simulink model "station_no_recovery"  (R2015a)
settings: Solver=ode45  StartTime=0  StopTime=5000  FixedStep=10  MaxStep=1  RelTol=1e-3
(part 4 of 4)

== system station_no_recovery/Восстанавливаемые объекты/ПАЭС-2500/Subsystem2/Element Exponential1 ==
  note: интенсивность событий
      | в рассматриваемом потоке
  "lambda " : Inport
  t : Inport  Port=2
  Divide : Product  Inputs=**
  Gain : Gain  Gain=-1
  Math Function : Math  SaturateOnIntegerOverflow=on
  P(t)1 : Outport
  wires:
  "lambda "/1 -> Divide/2
  Math Function/1 -> P(t)1/1
  Gain/1 -> Math Function/1
  t/1 -> Divide/1
  Divide/1 -> Gain/1

== system station_no_recovery/Восстанавливаемые объекты/ПАЭС-2500/Subsystem2/Element Normal ==
  note: математическое ожидание
      | наработки до отказа
  note: среднее квадратическое
      | отклонение наработки
      | до отказа
  "lambda " : Inport
  "M " : Inport  Port=2
  t : Inport  Port=3
  1-Q(t)1 : Fcn  Expr=1-u(1)
  MATLAB Function : MATLAB Function  TreatAsAtomicUnit=on
  P(t) : Outport
  wires:
  t/1 -> MATLAB Function/1(t)
  MATLAB Function/1(y) -> 1-Q(t)1/1
  "lambda "/1 -> MATLAB Function/2(sigma)
  1-Q(t)1/1 -> P(t)/1
  "M "/1 -> MATLAB Function/3(M)

== system station_no_recovery/Восстанавливаемые объекты/ПАЭС-2500/Subsystem2/Element Normal1 ==
  note: среднее квадратическое
      | отклонение наработки
      | до отказа
  note: математическое ожидание
      | наработки до отказа
  "lambda " : Inport
  "M " : Inport  Port=2
  t : Inport  Port=3
  1-Q(t)1 : Fcn  Expr=1-u(1)
  MATLAB Function : MATLAB Function  TreatAsAtomicUnit=on
  P(t) : Outport
  wires:
  "M "/1 -> MATLAB Function/3(M)
  1-Q(t)1/1 -> P(t)/1
  "lambda "/1 -> MATLAB Function/2(sigma)
  MATLAB Function/1(y) -> 1-Q(t)1/1
  t/1 -> MATLAB Function/1(t)

== system station_no_recovery/Восстанавливаемые объекты/ПАЭС-2500/Subsystem2/Сircuit Series ==
  P1 : Inport
  P2 : Inport  Port=2
  Fcn : Fcn  Expr=u(1)*u(2)
  Mux : Mux  Inputs=2
  P12 : Outport
  wires:
  Mux/1 -> Fcn/1
  P1/1 -> Mux/1
  Fcn/1 -> P12/1
  P2/1 -> Mux/2

== system station_no_recovery/Восстанавливаемые объекты/ПАЭС-2500/Subsystem2/Сircuit Series1 ==
  P1 : Inport
  P2 : Inport  Port=2
  Fcn : Fcn  Expr=u(1)*u(2)
  Mux : Mux  Inputs=2
  P12 : Outport
  wires:
  P2/1 -> Mux/2
  Fcn/1 -> P12/1
  P1/1 -> Mux/1
  Mux/1 -> Fcn/1

== system station_no_recovery/Восстанавливаемые объекты/ПАЭС-2500/Subsystem3/Element Exponential ==
  note: интенсивность событий
      | в рассматриваемом потоке
  "lambda " : Inport
  t : Inport  Port=2
  Divide : Product  Inputs=**
  Gain : Gain  Gain=-1
  Math Function : Math  SaturateOnIntegerOverflow=on
  P(t)1 : Outport
  wires:
  "lambda "/1 -> Divide/2
  Math Function/1 -> P(t)1/1
  Gain/1 -> Math Function/1
  t/1 -> Divide/1
  Divide/1 -> Gain/1

== system station_no_recovery/Восстанавливаемые объекты/ПАЭС-2500/Subsystem3/Element Exponential1 ==
  note: интенсивность событий
      | в рассматриваемом потоке
  "lambda " : Inport
  t : Inport  Port=2
  Divide : Product  Inputs=**
  Gain : Gain  Gain=-1
  Math Function : Math  SaturateOnIntegerOverflow=on
  P(t)1 : Outport
  wires:
  Divide/1 -> Gain/1
  t/1 -> Divide/1
  Gain/1 -> Math Function/1
  Math Function/1 -> P(t)1/1
  "lambda "/1 -> Divide/2

== system station_no_recovery/Восстанавливаемые объекты/ПАЭС-2500/Subsystem3/Element Normal ==
  note: среднее квадратическое
      | отклонение наработки
      | до отказа
  note: математическое ожидание
      | наработки до отказа
  "lambda " : Inport
  "M " : Inport  Port=2
  t : Inport  Port=3
  1-Q(t)1 : Fcn  Expr=1-u(1)
  MATLAB Function : MATLAB Function  TreatAsAtomicUnit=on
  P(t) : Outport
  wires:
  "M "/1 -> MATLAB Function/3(M)
  1-Q(t)1/1 -> P(t)/1
  "lambda "/1 -> MATLAB Function/2(sigma)
  MATLAB Function/1(y) -> 1-Q(t)1/1
  t/1 -> MATLAB Function/1(t)

== system station_no_recovery/Восстанавливаемые объекты/ПАЭС-2500/Subsystem3/Element Normal1 ==
  note: математическое ожидание
      | наработки до отказа
  note: среднее квадратическое
      | отклонение наработки
      | до отказа
  "lambda " : Inport
  "M " : Inport  Port=2
  t : Inport  Port=3
  1-Q(t)1 : Fcn  Expr=1-u(1)
  MATLAB Function : MATLAB Function  TreatAsAtomicUnit=on
  P(t) : Outport
  wires:
  t/1 -> MATLAB Function/1(t)
  MATLAB Function/1(y) -> 1-Q(t)1/1
  "lambda "/1 -> MATLAB Function/2(sigma)
  1-Q(t)1/1 -> P(t)/1
  "M "/1 -> MATLAB Function/3(M)

== system station_no_recovery/Восстанавливаемые объекты/ПАЭС-2500/Subsystem3/Сircuit Series ==
  P1 : Inport
  P2 : Inport  Port=2
  Fcn : Fcn  Expr=u(1)*u(2)
  Mux : Mux  Inputs=2
  P12 : Outport
  wires:
  P2/1 -> Mux/2
  Fcn/1 -> P12/1
  P1/1 -> Mux/1
  Mux/1 -> Fcn/1

== system station_no_recovery/Восстанавливаемые объекты/ПАЭС-2500/Subsystem3/Сircuit Series1 ==
  P1 : Inport
  P2 : Inport  Port=2
  Fcn : Fcn  Expr=u(1)*u(2)
  Mux : Mux  Inputs=2
  P12 : Outport
  wires:
  Mux/1 -> Fcn/1
  P1/1 -> Mux/1
  Fcn/1 -> P12/1
  P2/1 -> Mux/2

== system station_no_recovery/Восстанавливаемые объекты/САТУРН/Subsystem1/Element Exponential ==
  note: интенсивность событий
      | в рассматриваемом потоке
  "lambda " : Inport
  t : Inport  Port=2
  Divide : Product  Inputs=**
  Gain : Gain  Gain=-1
  Math Function : Math  SaturateOnIntegerOverflow=on
  P(t)1 : Outport
  wires:
  Divide/1 -> Gain/1
  t/1 -> Divide/1
  Gain/1 -> Math Function/1
  Math Function/1 -> P(t)1/1
  "lambda "/1 -> Divide/2

== system station_no_recovery/Восстанавливаемые объекты/САТУРН/Subsystem1/Element Normal ==
  note: математическое ожидание
      | наработки до отказа
  note: среднее квадратическое
      | отклонение наработки
      | до отказа
  "lambda " : Inport
  "M " : Inport  Port=2
  t : Inport  Port=3
  1-Q(t)1 : Fcn  Expr=1-u(1)
  MATLAB Function : MATLAB Function  TreatAsAtomicUnit=on
  P(t) : Outport
  wires:
  t/1 -> MATLAB Function/1(t)
  MATLAB Function/1(y) -> 1-Q(t)1/1
  "lambda "/1 -> MATLAB Function/2(sigma)
  1-Q(t)1/1 -> P(t)/1
  "M "/1 -> MATLAB Function/3(M)

== system station_no_recovery/Восстанавливаемые объекты/САТУРН/Subsystem1/Сircuit Series ==
  P1 : Inport
  P2 : Inport  Port=2
  Fcn : Fcn  Expr=u(1)*u(2)
  Mux : Mux  Inputs=2
  P12 : Outport
  wires:
  Mux/1 -> Fcn/1
  P1/1 -> Mux/1
  Fcn/1 -> P12/1
  P2/1 -> Mux/2

== system station_no_recovery/Восстанавливаемые объекты/САТУРН/Subsystem2/Element Exponential ==
  note: интенсивность событий
      | в рассматриваемом потоке
  "lambda " : Inport
  t : Inport  Port=2
  Divide : Product  Inputs=**
  Gain : Gain  Gain=-1
  Math Function : Math  SaturateOnIntegerOverflow=on
  P(t)1 : Outport
  wires:
  "lambda "/1 -> Divide/2
  Math Function/1 -> P(t)1/1
  Gain/1 -> Math Function/1
  t/1 -> Divide/1
  Divide/1 -> Gain/1

== system station_no_recovery/Восстанавливаемые объекты/САТУРН/Subsystem2/Element Normal ==
  note: среднее квадратическое
      | отклонение наработки
      | до отказа
  note: математическое ожидание
      | наработки до отказа
  "lambda " : Inport
  "M " : Inport  Port=2
  t : Inport  Port=3
  1-Q(t)1 : Fcn  Expr=1-u(1)
  MATLAB Function : MATLAB Function  TreatAsAtomicUnit=on
  P(t) : Outport
  wires:
  "M "/1 -> MATLAB Function/3(M)
  1-Q(t)1/1 -> P(t)/1
  "lambda "/1 -> MATLAB Function/2(sigma)
  MATLAB Function/1(y) -> 1-Q(t)1/1
  t/1 -> MATLAB Function/1(t)

== system station_no_recovery/Восстанавливаемые объекты/САТУРН/Subsystem2/Сircuit Series ==
  P1 : Inport
  P2 : Inport  Port=2
  Fcn : Fcn  Expr=u(1)*u(2)
  Mux : Mux  Inputs=2
  P12 : Outport
  wires:
  P2/1 -> Mux/2
  Fcn/1 -> P12/1
  P1/1 -> Mux/1
  Mux/1 -> Fcn/1

== system station_no_recovery/Восстанавливаемые объекты/САТУРН/Subsystem3/Element Exponential ==
  note: интенсивность событий
      | в рассматриваемом потоке
  "lambda " : Inport
  t : Inport  Port=2
  Divide : Product  Inputs=**
  Gain : Gain  Gain=-1
  Math Function : Math  SaturateOnIntegerOverflow=on
  P(t)1 : Outport
  wires:
  Divide/1 -> Gain/1
  t/1 -> Divide/1
  Gain/1 -> Math Function/1
  Math Function/1 -> P(t)1/1
  "lambda "/1 -> Divide/2

== system station_no_recovery/Восстанавливаемые объекты/САТУРН/Subsystem3/Element Normal ==
  note: математическое ожидание
      | наработки до отказа
  note: среднее квадратическое
      | отклонение наработки
      | до отказа
  "lambda " : Inport
  "M " : Inport  Port=2
  t : Inport  Port=3
  1-Q(t)1 : Fcn  Expr=1-u(1)
  MATLAB Function : MATLAB Function  TreatAsAtomicUnit=on
  P(t) : Outport
  wires:
  t/1 -> MATLAB Function/1(t)
  MATLAB Function/1(y) -> 1-Q(t)1/1
  "lambda "/1 -> MATLAB Function/2(sigma)
  1-Q(t)1/1 -> P(t)/1
  "M "/1 -> MATLAB Function/3(M)

== system station_no_recovery/Восстанавливаемые объекты/САТУРН/Subsystem3/Сircuit Series ==
  P1 : Inport
  P2 : Inport  Port=2
  Fcn : Fcn  Expr=u(1)*u(2)
  Mux : Mux  Inputs=2
  P12 : Outport
  wires:
  Mux/1 -> Fcn/1
  P1/1 -> Mux/1
  Fcn/1 -> P12/1
  P2/1 -> Mux/2

== system station_no_recovery/Восстанавливаемые объекты/САТУРН/Subsystem4/Element Exponential ==
  note: интенсивность событий
      | в рассматриваемом потоке
  "lambda " : Inport
  t : Inport  Port=2
  Divide : Product  Inputs=**
  Gain : Gain  Gain=-1
  Math Function : Math  SaturateOnIntegerOverflow=on
  P(t)1 : Outport
  wires:
  "lambda "/1 -> Divide/2
  Math Function/1 -> P(t)1/1
  Gain/1 -> Math Function/1
  t/1 -> Divide/1
  Divide/1 -> Gain/1

== system station_no_recovery/Восстанавливаемые объекты/САТУРН/Subsystem4/Element Normal ==
  note: среднее квадратическое
      | отклонение наработки
      | до отказа
  note: математическое ожидание
      | наработки до отказа
  "lambda " : Inport
  "M " : Inport  Port=2
  t : Inport  Port=3
  1-Q(t)1 : Fcn  Expr=1-u(1)
  MATLAB Function : MATLAB Function  TreatAsAtomicUnit=on
  P(t) : Outport
  wires:
  "M "/1 -> MATLAB Function/3(M)
  1-Q(t)1/1 -> P(t)/1
  "lambda "/1 -> MATLAB Function/2(sigma)
  MATLAB Function/1(y) -> 1-Q(t)1/1
  t/1 -> MATLAB Function/1(t)

== system station_no_recovery/Восстанавливаемые объекты/САТУРН/Subsystem4/Сircuit Series ==
  P1 : Inport
  P2 : Inport  Port=2
  Fcn : Fcn  Expr=u(1)*u(2)
  Mux : Mux  Inputs=2
  P12 : Outport
  wires:
  P2/1 -> Mux/2
  Fcn/1 -> P12/1
  P1/1 -> Mux/1
  Mux/1 -> Fcn/1

== system station_no_recovery/Восстанавливаемые объекты/УРАЛ-6000/Subsystem1/Element Exponential ==
  note: интенсивность событий
      | в рассматриваемом потоке
  "lambda " : Inport
  t : Inport  Port=2
  Divide : Product  Inputs=**
  Gain : Gain  Gain=-1
  Math Function : Math  SaturateOnIntegerOverflow=on
  P(t)1 : Outport
  wires:
  Divide/1 -> Gain/1
  t/1 -> Divide/1
  Gain/1 -> Math Function/1
  Math Function/1 -> P(t)1/1
  "lambda "/1 -> Divide/2

== system station_no_recovery/Восстанавливаемые объекты/УРАЛ-6000/Subsystem1/Element Normal ==
  note: математическое ожидание
      | наработки до отказа
  note: среднее квадратическое
      | отклонение наработки
      | до отказа
  "lambda " : Inport
  "M " : Inport  Port=2
  t : Inport  Port=3
  1-Q(t)1 : Fcn  Expr=1-u(1)
  MATLAB Function : MATLAB Function  TreatAsAtomicUnit=on
  P(t) : Outport
  wires:
  t/1 -> MATLAB Function/1(t)
  MATLAB Function/1(y) -> 1-Q(t)1/1
  "lambda "/1 -> MATLAB Function/2(sigma)
  1-Q(t)1/1 -> P(t)/1
  "M "/1 -> MATLAB Function/3(M)

== system station_no_recovery/Восстанавливаемые объекты/УРАЛ-6000/Subsystem1/Сircuit Series ==
  P1 : Inport
  P2 : Inport  Port=2
  Fcn : Fcn  Expr=u(1)*u(2)
  Mux : Mux  Inputs=2
  P12 : Outport
  wires:
  Mux/1 -> Fcn/1
  P1/1 -> Mux/1
  Fcn/1 -> P12/1
  P2/1 -> Mux/2

== system station_no_recovery/Восстанавливаемые объекты/УРАЛ-6000/Subsystem2/Element Exponential ==
  note: интенсивность событий
      | в рассматриваемом потоке
  "lambda " : Inport
  t : Inport  Port=2
  Divide : Product  Inputs=**
  Gain : Gain  Gain=-1
  Math Function : Math  SaturateOnIntegerOverflow=on
  P(t)1 : Outport
  wires:
  "lambda "/1 -> Divide/2
  Math Function/1 -> P(t)1/1
  Gain/1 -> Math Function/1
  t/1 -> Divide/1
  Divide/1 -> Gain/1

== system station_no_recovery/Восстанавливаемые объекты/УРАЛ-6000/Subsystem2/Element Normal ==
  note: среднее квадратическое
      | отклонение наработки
      | до отказа
  note: математическое ожидание
      | наработки до отказа
  "lambda " : Inport
  "M " : Inport  Port=2
  t : Inport  Port=3
  1-Q(t)1 : Fcn  Expr=1-u(1)
  MATLAB Function : MATLAB Function  TreatAsAtomicUnit=on
  P(t) : Outport
  wires:
  "M "/1 -> MATLAB Function/3(M)
  1-Q(t)1/1 -> P(t)/1
  "lambda "/1 -> MATLAB Function/2(sigma)
  MATLAB Function/1(y) -> 1-Q(t)1/1
  t/1 -> MATLAB Function/1(t)

== system station_no_recovery/Восстанавливаемые объекты/УРАЛ-6000/Subsystem2/Сircuit Series ==
  P1 : Inport
  P2 : Inport  Port=2
  Fcn : Fcn  Expr=u(1)*u(2)
  Mux : Mux  Inputs=2
  P12 : Outport
  wires:
  P2/1 -> Mux/2
  Fcn/1 -> P12/1
  P1/1 -> Mux/1
  Mux/1 -> Fcn/1

== system station_no_recovery/Восстанавливаемые объекты/УРАЛ-6000/Subsystem3/Element Exponential ==
  note: интенсивность событий
      | в рассматриваемом потоке
  "lambda " : Inport
  t : Inport  Port=2
  Divide : Product  Inputs=**
  Gain : Gain  Gain=-1
  Math Function : Math  SaturateOnIntegerOverflow=on
  P(t)1 : Outport
  wires:
  "lambda "/1 -> Divide/2
  Math Function/1 -> P(t)1/1
  Gain/1 -> Math Function/1
  t/1 -> Divide/1
  Divide/1 -> Gain/1

== system station_no_recovery/Восстанавливаемые объекты/УРАЛ-6000/Subsystem3/Element Normal ==
  note: среднее квадратическое
      | отклонение наработки
      | до отказа
  note: математическое ожидание
      | наработки до отказа
  "lambda " : Inport
  "M " : Inport  Port=2
  t : Inport  Port=3
  1-Q(t)1 : Fcn  Expr=1-u(1)
  MATLAB Function : MATLAB Function  TreatAsAtomicUnit=on
  P(t) : Outport
  wires:
  "M "/1 -> MATLAB Function/3(M)
  1-Q(t)1/1 -> P(t)/1
  "lambda "/1 -> MATLAB Function/2(sigma)
  MATLAB Function/1(y) -> 1-Q(t)1/1
  t/1 -> MATLAB Function/1(t)

== system station_no_recovery/Восстанавливаемые объекты/УРАЛ-6000/Subsystem3/Сircuit Series ==
  P1 : Inport
  P2 : Inport  Port=2
  Fcn : Fcn  Expr=u(1)*u(2)
  Mux : Mux  Inputs=2
  P12 : Outport
  wires:
  P2/1 -> Mux/2
  Fcn/1 -> P12/1
  P1/1 -> Mux/1
  Mux/1 -> Fcn/1

== system station_no_recovery/Восстанавливаемые объекты/УРАЛ-6000/Subsystem4/Element Exponential ==
  note: интенсивность событий
      | в рассматриваемом потоке
  "lambda " : Inport
  t : Inport  Port=2
  Divide : Product  Inputs=**
  Gain : Gain  Gain=-1
  Math Function : Math  SaturateOnIntegerOverflow=on
  P(t)1 : Outport
  wires:
  Divide/1 -> Gain/1
  t/1 -> Divide/1
  Gain/1 -> Math Function/1
  Math Function/1 -> P(t)1/1
  "lambda "/1 -> Divide/2

== system station_no_recovery/Восстанавливаемые объекты/УРАЛ-6000/Subsystem4/Element Normal ==
  note: математическое ожидание
      | наработки до отказа
  note: среднее квадратическое
      | отклонение наработки
      | до отказа
  "lambda " : Inport
  "M " : Inport  Port=2
  t : Inport  Port=3
  1-Q(t)1 : Fcn  Expr=1-u(1)
  MATLAB Function : MATLAB Function  TreatAsAtomicUnit=on
  P(t) : Outport
  wires:
  t/1 -> MATLAB Function/1(t)
  MATLAB Function/1(y) -> 1-Q(t)1/1
  "lambda "/1 -> MATLAB Function/2(sigma)
  1-Q(t)1/1 -> P(t)/1
  "M "/1 -> MATLAB Function/3(M)

== system station_no_recovery/Восстанавливаемые объекты/УРАЛ-6000/Subsystem4/Сircuit Series ==
  P1 : Inport
  P2 : Inport  Port=2
  Fcn : Fcn  Expr=u(1)*u(2)
  Mux : Mux  Inputs=2
  P12 : Outport
  wires:
  Mux/1 -> Fcn/1
  P1/1 -> Mux/1
  Fcn/1 -> P12/1
  P2/1 -> Mux/2

== system station_no_recovery/Восстанавливаемые объекты/ЭГ-12/Subsystem1/Element Exponential ==
  note: интенсивность событий
      | в рассматриваемом потоке
  "lambda " : Inport
  t : Inport  Port=2
  Divide : Product  Inputs=**
  Gain : Gain  Gain=-1
  Math Function : Math  SaturateOnIntegerOverflow=on
  P(t)1 : Outport
  wires:
  "lambda "/1 -> Divide/2
  Math Function/1 -> P(t)1/1
  Gain/1 -> Math Function/1
  t/1 -> Divide/1
  Divide/1 -> Gain/1

== system station_no_recovery/Восстанавливаемые объекты/ЭГ-12/Subsystem1/Element Normal ==
  note: среднее квадратическое
      | отклонение наработки
      | до отказа
  note: математическое ожидание
      | наработки до отказа
  "lambda " : Inport
  "M " : Inport  Port=2
  t : Inport  Port=3
  1-Q(t)1 : Fcn  Expr=1-u(1)
  MATLAB Function : MATLAB Function  TreatAsAtomicUnit=on
  P(t) : Outport
  wires:
  "M "/1 -> MATLAB Function/3(M)
  1-Q(t)1/1 -> P(t)/1
  "lambda "/1 -> MATLAB Function/2(sigma)
  MATLAB Function/1(y) -> 1-Q(t)1/1
  t/1 -> MATLAB Function/1(t)

== system station_no_recovery/Восстанавливаемые объекты/ЭГ-12/Subsystem1/Сircuit Series ==
  P1 : Inport
  P2 : Inport  Port=2
  Fcn : Fcn  Expr=u(1)*u(2)
  Mux : Mux  Inputs=2
  P12 : Outport
  wires:
  P2/1 -> Mux/2
  Fcn/1 -> P12/1
  P1/1 -> Mux/1
  Mux/1 -> Fcn/1

== system station_no_recovery/Восстанавливаемые объекты/ЭГ-12/Subsystem3/Element Exponential ==
  note: интенсивность событий
      | в рассматриваемом потоке
  "lambda " : Inport
  t : Inport  Port=2
  Divide : Product  Inputs=**
  Gain : Gain  Gain=-1
  Math Function : Math  SaturateOnIntegerOverflow=on
  P(t)1 : Outport
  wires:
  Divide/1 -> Gain/1
  t/1 -> Divide/1
  Gain/1 -> Math Function/1
  Math Function/1 -> P(t)1/1
  "lambda "/1 -> Divide/2

== system station_no_recovery/Восстанавливаемые объекты/ЭГ-12/Subsystem3/Element Normal ==
  note: математическое ожидание
      | наработки до отказа
  note: среднее квадратическое
      | отклонение наработки
      | до отказа
  "lambda " : Inport
  "M " : Inport  Port=2
  t : Inport  Port=3
  1-Q(t)1 : Fcn  Expr=1-u(1)
  MATLAB Function : MATLAB Function  TreatAsAtomicUnit=on
  P(t) : Outport
  wires:
  t/1 -> MATLAB Function/1(t)
  MATLAB Function/1(y) -> 1-Q(t)1/1
  "lambda "/1 -> MATLAB Function/2(sigma)
  1-Q(t)1/1 -> P(t)/1
  "M "/1 -> MATLAB Function/3(M)

== system station_no_recovery/Восстанавливаемые объекты/ЭГ-12/Subsystem3/Сircuit Series ==
  P1 : Inport
  P2 : Inport  Port=2
  Fcn : Fcn  Expr=u(1)*u(2)
  Mux : Mux  Inputs=2
  P12 : Outport
  wires:
  Mux/1 -> Fcn/1
  P1/1 -> Mux/1
  Fcn/1 -> P12/1
  P2/1 -> Mux/2

== matlab function station_no_recovery/Восстанавливаемые объекты/ПАЭС-2500/Subsystem/Element Normal1/MATLAB Function ==
  data: t input; y output; sigma input; M input
function y = fcn(t,sigma,M)
y=normcdf((t-M)/sigma);

== matlab function station_no_recovery/Восстанавливаемые объекты/ГТЭ-6//6,3/Subsystem1/Element Normal/MATLAB Function ==
  data: t input; y output; sigma input; M input
function y = fcn(t,sigma,M)
y=normcdf((t-M)/sigma);

== stateflow chart station_no_recovery/Восстанавливаемые объекты/ПАЭС-2500/Subsystem1/Chart ==
  note: Параметры:
      | Входные:
      | dP - доля деградации при каждой итерации по вероятности
      | t - текущее время
      | Pz - заданная вероятность
      | P0 - вероятность, пересчитанная по времени
      | delta_t - время восстановления объекта
      | trec - время капитального ремонта
      | t_start - начальная выработка объекта
      |
      | Локальные:
      | i-количество восстановлений по вероятности(начинается с 0)
      | j-количество капитальных восстановлений (начинается с 1)
      | delta_P - dP * i
      | t0 - время, когда произошло восстановление (нужно для обнуления времени)
      | t_s = начальная выработка объекта (обнуляется после восстановления)
      |
      | Выходные:
      | tv - пересчитанное время
      | P - пересчитанная итоговая вероятность
  state repair
    entry:
    t0=t;
    tv=t-t0;
    P=0;
    during:
    P=0;
    tv=t-t0;
  state work
    entry:
    delta_P=dP*i;
    P=P0-delta_P;
    during:
    P=P0-delta_P;
    tv=t+t_s-t0;
  (default) -> work : {i=0; j=1; t0=0; t_s=t_start; P=1; tv=t_s;}
  work -> repair [order 1] : [P<=Pz]{i=i+1;t_s=0;}
  repair -> work : [t-t0>=delta_t]
  work -> repair [order 2] : [t+t_s>=trec*j]{j=j+1;t_s=0;i=0;}
  data: t_start input; delta_t input; Pz input; trec input; dP input; t input; tv output; P output; j local; delta_P local; t_s local; i local; t0 local; P0 input

== matlab function station_no_recovery/Восстанавливаемые объекты/УРАЛ-6000/Subsystem2/Element Normal/MATLAB Function ==
  data: t input; y output; sigma input; M input
function y = fcn(t,sigma,M)
y=normcdf((t-M)/sigma);

== matlab function station_no_recovery/Восстанавливаемые объекты/ПАЭС-2500/Subsystem1/Element Normal/MATLAB Function ==
  data: t input; y output; sigma input; M input
function y = fcn(t,sigma,M)
y=normcdf((t-M)/sigma);

== matlab function station_no_recovery/Восстанавливаемые объекты/ЭГ-12/Subsystem3/Element Normal/MATLAB Function ==
  data: t input; y output; sigma input; M input
function y = fcn(t,sigma,M)
y=normcdf((t-M)/sigma);

== stateflow chart station_no_recovery/Восстанавливаемые объекты/ГТЭ-6//6,3/Subsystem1/Chart ==
  note: Параметры:
      | Входные:
      | dP - доля деградации при каждой итерации по вероятности
      | t - текущее время
      | Pz - заданная вероятность
      | P0 - вероятность, пересчитанная по времени
      | delta_t - время восстановления объекта
      | trec - время капитального ремонта
      | t_start - начальная выработка объекта
      |
      | Локальные:
      | i-количество восстановлений по вероятности(начинается с 0)
      | j-количество капитальных восстановлений (начинается с 1)
      | delta_P - dP * i
      | t0 - время, когда произошло восстановление (нужно для обнуления времени)
      | t_s = начальная выработка объекта (обнуляется после восстановления)
      |
      | Выходные:
      | tv - пересчитанное время
      | P - пересчитанная итоговая вероятность
  state repair
    entry:
    t0=t;
    tv=t-t0;
    P=0;
    during:
    P=0;
    tv=t-t0;
  state work
    entry:
    delta_P=dP*i;
    P=P0-delta_P;
    during:
    P=P0-delta_P;
    tv=t+t_s-t0;
  (default) -> work : {i=0; j=1; t0=0; t_s=t_start; P=1; tv=t_s;}
  work -> repair [order 1] : [P<=Pz]{i=i+1;t_s=0;}
  repair -> work : [t-t0>=delta_t]
  work -> repair [order 2] : [t+t_s>=trec*j]{j=j+1;t_s=0;i=0;}
  data: t_start input; delta_t input; Pz input; trec input; dP input; t input; tv output; P output; j local; delta_P local; t_s local; i local; t0 local; P0 input

== matlab function station_no_recovery/Восстанавливаемые объекты/ПАЭС-2500/Subsystem/Element Normal/MATLAB Function ==
  data: t input; y output; sigma input; M input
function y = fcn(t,sigma,M)
y=normcdf((t-M)/sigma);

== matlab function station_no_recovery/Восстанавливаемые объекты/САТУРН/Subsystem4/Element Normal/MATLAB Function ==
  data: t input; y output; sigma input; M input
function y = fcn(t,sigma,M)
y=normcdf((t-M)/sigma);

== matlab function station_no_recovery/Схема/Сircuit n Parallel1/n Parallel Function ==
  data: Pn output; P input
function Pn = fcn(P)
[n,col]=size(P);
u=1;
for i=1:n
   u=u*(1-P(i)); 
end
Pn = 1 - u;

== matlab function station_no_recovery/Восстанавливаемые объекты/ПАЭС-2500/Subsystem1/Element Normal1/MATLAB Function ==
  data: t input; y output; sigma input; M input
function y = fcn(t,sigma,M)
y=normcdf((t-M)/sigma);

== stateflow chart station_no_recovery/Восстанавливаемые объекты/ПАЭС-2500/Subsystem/Chart ==
  note: Параметры:
      | Входные:
      | dP - доля деградации при каждой итерации по вероятности
      | t - текущее время
      | Pz - заданная вероятность
      | P0 - вероятность, пересчитанная по времени
      | delta_t - время восстановления объекта
      | trec - время капитального ремонта
      | t_start - начальная выработка объекта
      |
      | Локальные:
      | i-количество восстановлений по вероятности(начинается с 0)
      | j-количество капитальных восстановлений (начинается с 1)
      | delta_P - dP * i
      | t0 - время, когда произошло восстановление (нужно для обнуления времени)
      | t_s = начальная выработка объекта (обнуляется после восстановления)
      |
      | Выходные:
      | tv - пересчитанное время
      | P - пересчитанная итоговая вероятность
  state repair
    entry:
    t0=t;
    tv=t-t0;
    P=0;
    during:
    P=0;
    tv=t-t0;
  state work
    entry:
    delta_P=dP*i;
    P=P0-delta_P;
    during:
    P=P0-delta_P;
    tv=t+t_s-t0;
  (default) -> work : {i=0; j=1; t0=0; t_s=t_start; P=1; tv=t_s;}
  work -> repair [order 1] : [P<=Pz]{i=i+1;t_s=0;}
  repair -> work : [t-t0>=delta_t]
  work -> repair [order 2] : [t+t_s>=trec*j]{j=j+1;t_s=0;i=0;}
  data: t_start input; delta_t input; Pz input; trec input; dP input; t input; tv output; P output; j local; delta_P local; t_s local; i local; t0 local; P0 input

== stateflow chart station_no_recovery/Восстанавливаемые объекты/УРАЛ-6000/Subsystem2/Chart ==
  note: Параметры:
      | Входные:
      | dP - доля деградации при каждой итерации по вероятности
      | t - текущее время
      | Pz - заданная вероятность
      | P0 - вероятность, пересчитанная по времени
      | delta_t - время восстановления объекта
      | trec - время капитального ремонта
      | t_start - начальная выработка объекта
      |
      | Локальные:
      | i-количество восстановлений по вероятности(начинается с 0)
      | j-количество капитальных восстановлений (начинается с 1)
      | delta_P - dP * i
      | t0 - время, когда произошло восстановление (нужно для обнуления времени)
      | t_s = начальная выработка объекта (обнуляется после восстановления)
      |
      | Выходные:
      | tv - пересчитанное время
      | P - пересчитанная итоговая вероятность
  state repair
    entry:
    t0=t;
    tv=t-t0;
    P=0;
    during:
    P=0;
    tv=t-t0;
  state work
    entry:
    delta_P=dP*i;
    P=P0-delta_P;
    during:
    P=P0-delta_P;
    tv=t+t_s-t0;
  (default) -> work : {i=0; j=1; t0=0; t_s=t_start; P=1; tv=t_s;}
  work -> repair [order 1] : [P<=Pz]{i=i+1;t_s=0;}
  repair -> work : [t-t0>=delta_t]
  work -> repair [order 2] : [t+t_s>=trec*j]{j=j+1;t_s=0;i=0;}
  data: t_start input; delta_t input; Pz input; trec input; dP input; t input; tv output; P output; j local; delta_P local; t_s local; i local; t0 local; P0 input

== stateflow chart station_no_recovery/Восстанавливаемые объекты/ЭГ-12/Subsystem3/Chart ==
  note: Параметры:
      | Входные:
      | dP - доля деградации при каждой итерации по вероятности
      | t - текущее время
      | Pz - заданная вероятность
      | P0 - вероятность, пересчитанная по времени
      | delta_t - время восстановления объекта
      | trec - время капитального ремонта
      | t_start - начальная выработка объекта
      |
      | Локальные:
      | i-количество восстановлений по вероятности(начинается с 0)
      | j-количество капитальных восстановлений (начинается с 1)
      | delta_P - dP * i
      | t0 - время, когда произошло восстановление (нужно для обнуления времени)
      | t_s = начальная выработка объекта (обнуляется после восстановления)
      |
      | Выходные:
      | tv - пересчитанное время
      | P - пересчитанная итоговая вероятность
  state repair
    entry:
    t0=t;
    tv=t-t0;
    P=0;
    during:
    P=0;
    tv=t-t0;
  state work
    entry:
    delta_P=dP*i;
    P=P0-delta_P;
    during:
    P=P0-delta_P;
    tv=t+t_s-t0;
  (default) -> work : {i=0; j=1; t0=0; t_s=t_start; P=1; tv=t_s;}
  work -> repair [order 1] : [P<=Pz]{i=i+1;t_s=0;}
  repair -> work : [t-t0>=delta_t]
  work -> repair [order 2] : [t+t_s>=trec*j]{j=j+1;t_s=0;i=0;}
  data: t_start input; delta_t input; Pz input; trec input; dP input; t input; tv output; P output; j local; delta_P local; t_s local; i local; t0 local; P0 input

== stateflow chart station_no_recovery/Восстанавливаемые объекты/САТУРН/Subsystem4/Chart ==
  note: Параметры:
      | Входные:
      | dP - доля деградации при каждой итерации по вероятности
      | t - текущее время
      | Pz - заданная вероятность
      | P0 - вероятность, пересчитанная по времени
      | delta_t - время восстановления объекта
      | trec - время капитального ремонта
      | t_start - начальная выработка объекта
      |
      | Локальные:
      | i-количество восстановлений по вероятности(начинается с 0)
      | j-количество капитальных восстановлений (начинается с 1)
      | delta_P - dP * i
      | t0 - время, когда произошло восстановление (нужно для обнуления времени)
      | t_s = начальная выработка объекта (обнуляется после восстановления)
      |
      | Выходные:
      | tv - пересчитанное время
      | P - пересчитанная итоговая вероятность
  state repair
    entry:
    t0=t;
    tv=t-t0;
    P=0;
    during:
    P=0;
    tv=t-t0;
  state work
    entry:
    delta_P=dP*i;
    P=P0-delta_P;
    during:
    P=P0-delta_P;
    tv=t+t_s-t0;
  (default) -> work : {i=0; j=1; t0=0; t_s=t_start; P=1; tv=t_s;}
  work -> repair [order 1] : [P<=Pz]{i=i+1;t_s=0;}
  repair -> work : [t-t0>=delta_t]
  work -> repair [order 2] : [t+t_s>=trec*j]{j=j+1;t_s=0;i=0;}
  data: t_start input; delta_t input; Pz input; trec input; dP input; t input; tv output; P output; j local; delta_P local; t_s local; i local; t0 local; P0 input

== stateflow chart station_no_recovery/Восстанавливаемые объекты/ПАЭС-2500/Subsystem2/Chart ==
  note: Параметры:
      | Входные:
      | dP - доля деградации при каждой итерации по вероятности
      | t - текущее время
      | Pz - заданная вероятность
      | P0 - вероятность, пересчитанная по времени
      | delta_t - время восстановления объекта
      | trec - время капитального ремонта
      | t_start - начальная выработка объекта
      |
      | Локальные:
      | i-количество восстановлений по вероятности(начинается с 0)
      | j-количество капитальных восстановлений (начинается с 1)
      | delta_P - dP * i
      | t0 - время, когда произошло восстановление (нужно для обнуления времени)
      | t_s = начальная выработка объекта (обнуляется после восстановления)
      |
      | Выходные:
      | tv - пересчитанное время
      | P - пересчитанная итоговая вероятность
  state repair
    entry:
    t0=t;
    tv=t-t0;
    P=0;
    during:
    P=0;
    tv=t-t0;
  state work
    entry:
    delta_P=dP*i;
    P=P0-delta_P;
    during:
    P=P0-delta_P;
    tv=t+t_s-t0;
  (default) -> work : {i=0; j=1; t0=0; t_s=t_start; P=1; tv=t_s;}
  work -> repair [order 1] : [P<=Pz]{i=i+1;t_s=0;}
  repair -> work : [t-t0>=delta_t]
  work -> repair [order 2] : [t+t_s>=trec*j]{j=j+1;t_s=0;i=0;}
  data: t_start input; delta_t input; Pz input; trec input; dP input; t input; tv output; P output; j local; delta_P local; t_s local; i local; t0 local; P0 input

== matlab function station_no_recovery/Восстанавливаемые объекты/ПАЭС-2500/Subsystem2/Element Normal/MATLAB Function ==
  data: t input; y output; sigma input; M input
function y = fcn(t,sigma,M)
y=normcdf((t-M)/sigma);

== matlab function station_no_recovery/Восстанавливаемые объекты/ПАЭС-2500/Subsystem2/Element Normal1/MATLAB Function ==
  data: t input; y output; sigma input; M input
function y = fcn(t,sigma,M)
y=normcdf((t-M)/sigma);

== stateflow chart station_no_recovery/Восстанавливаемые объекты/ПАЭС-2500/Subsystem3/Chart ==
  note: Параметры:
      | Входные:
      | dP - доля деградации при каждой итерации по вероятности
      | t - текущее время
      | Pz - заданная вероятность
      | P0 - вероятность, пересчитанная по времени
      | delta_t - время восстановления объекта
      | trec - время капитального ремонта
      | t_start - начальная выработка объекта
      |
      | Локальные:
      | i-количество восстановлений по вероятности(начинается с 0)
      | j-количество капитальных восстановлений (начинается с 1)
      | delta_P - dP * i
      | t0 - время, когда произошло восстановление (нужно для обнуления времени)
      | t_s = начальная выработка объекта (обнуляется после восстановления)
      |
      | Выходные:
      | tv - пересчитанное время
      | P - пересчитанная итоговая вероятность
  state repair
    entry:
    t0=t;
    tv=t-t0;
    P=0;
    during:
    P=0;
    tv=t-t0;
  state work
    entry:
    delta_P=dP*i;
    P=P0-delta_P;
    during:
    P=P0-delta_P;
    tv=t+t_s-t0;
  (default) -> work : {i=0; j=1; t0=0; t_s=t_start; P=1; tv=t_s;}
  work -> repair [order 1] : [P<=Pz]{i=i+1;t_s=0;}
  repair -> work : [t-t0>=delta_t]
  work -> repair [order 2] : [t+t_s>=trec*j]{j=j+1;t_s=0;i=0;}
  data: t_start input; delta_t input; Pz input; trec input; dP input; t input; tv output; P output; j local; delta_P local; t_s local; i local; t0 local; P0 input

== matlab function station_no_recovery/Восстанавливаемые объекты/ПАЭС-2500/Subsystem3/Element Normal/MATLAB Function ==
  data: t input; y output; sigma input; M input
function y = fcn(t,sigma,M)
y=normcdf((t-M)/sigma);

== matlab function station_no_recovery/Восстанавливаемые объекты/ПАЭС-2500/Subsystem3/Element Normal1/MATLAB Function ==
  data: t input; y output; sigma input; M input
function y = fcn(t,sigma,M)
y=normcdf((t-M)/sigma);

== stateflow chart station_no_recovery/Восстанавливаемые объекты/УРАЛ-6000/Subsystem1/Chart ==
  note: Параметры:
      | Входные:
      | dP - доля деградации при каждой итерации по вероятности
      | t - текущее время
      | Pz - заданная вероятность
      | P0 - вероятность, пересчитанная по времени
      | delta_t - время восстановления объекта
      | trec - время капитального ремонта
      | t_start - начальная выработка объекта
      |
      | Локальные:
      | i-количество восстановлений по вероятности(начинается с 0)
      | j-количество капитальных восстановлений (начинается с 1)
      | delta_P - dP * i
      | t0 - время, когда произошло восстановление (нужно для обнуления времени)
      | t_s = начальная выработка объекта (обнуляется после восстановления)
      |
      | Выходные:
      | tv - пересчитанное время
      | P - пересчитанная итоговая вероятность
  state repair
    entry:
    t0=t;
    tv=t-t0;
    P=0;
    during:
    P=0;
    tv=t-t0;
  state work
    entry:
    delta_P=dP*i;
    P=P0-delta_P;
    during:
    P=P0-delta_P;
    tv=t+t_s-t0;
  (default) -> work : {i=0; j=1; t0=0; t_s=t_start; P=1; tv=t_s;}
  work -> repair [order 1] : [P<=Pz]{i=i+1;t_s=0;}
  repair -> work : [t-t0>=delta_t]
  work -> repair [order 2] : [t+t_s>=trec*j]{j=j+1;t_s=0;i=0;}
  data: t_start input; delta_t input; Pz input; trec input; dP input; t input; tv output; P output; j local; delta_P local; t_s local; i local; t0 local; P0 input

== matlab function station_no_recovery/Восстанавливаемые объекты/УРАЛ-6000/Subsystem1/Element Normal/MATLAB Function ==
  data: t input; y output; sigma input; M input
function y = fcn(t,sigma,M)
y=normcdf((t-M)/sigma);

== stateflow chart station_no_recovery/Восстанавливаемые объекты/УРАЛ-6000/Subsystem3/Chart ==
  note: Параметры:
      | Входные:
      | dP - доля деградации при каждой итерации по вероятности
      | t - текущее время
      | Pz - заданная вероятность
      | P0 - вероятность, пересчитанная по времени
      | delta_t - время восстановления объекта
      | trec - время капитального ремонта
      | t_start - начальная выработка объекта
      |
      | Локальные:
      | i-количество восстановлений по вероятности(начинается с 0)
      | j-количество капитальных восстановлений (начинается с 1)
      | delta_P - dP * i
      | t0 - время, когда произошло восстановление (нужно для обнуления времени)
      | t_s = начальная выработка объекта (обнуляется после восстановления)
      |
      | Выходные:
      | tv - пересчитанное время
      | P - пересчитанная итоговая вероятность
  state repair
    entry:
    t0=t;
    tv=t-t0;
    P=0;
    during:
    P=0;
    tv=t-t0;
  state work
    entry:
    delta_P=dP*i;
    P=P0-delta_P;
    during:
    P=P0-delta_P;
    tv=t+t_s-t0;
  (default) -> work : {i=0; j=1; t0=0; t_s=t_start; P=1; tv=t_s;}
  work -> repair [order 1] : [P<=Pz]{i=i+1;t_s=0;}
  repair -> work : [t-t0>=delta_t]
  work -> repair [order 2] : [t+t_s>=trec*j]{j=j+1;t_s=0;i=0;}
  data: t_start input; delta_t input; Pz input; trec input; dP input; t input; tv output; P output; j local; delta_P local; t_s local; i local; t0 local; P0 input

== matlab function station_no_recovery/Восстанавливаемые объекты/УРАЛ-6000/Subsystem3/Element Normal/MATLAB Function ==
  data: t input; y output; sigma input; M input
function y = fcn(t,sigma,M)
y=normcdf((t-M)/sigma);

== stateflow chart station_no_recovery/Восстанавливаемые объекты/УРАЛ-6000/Subsystem4/Chart ==
  note: Параметры:
      | Входные:
      | dP - доля деградации при каждой итерации по вероятности
      | t - текущее время
      | Pz - заданная вероятность
      | P0 - вероятность, пересчитанная по времени
      | delta_t - время восстановления объекта
      | trec - время капитального ремонта
      | t_start - начальная выработка объекта
      |
      | Локальные:
      | i-количество восстановлений по вероятности(начинается с 0)
      | j-количество капитальных восстановлений (начинается с 1)
      | delta_P - dP * i
      | t0 - время, когда произошло восстановление (нужно для обнуления времени)
      | t_s = начальная выработка объекта (обнуляется после восстановления)
      |
      | Выходные:
      | tv - пересчитанное время
      | P - пересчитанная итоговая вероятность
  state repair
    entry:
    t0=t;
    tv=t-t0;
    P=0;
    during:
    P=0;
    tv=t-t0;
  state work
    entry:
    delta_P=dP*i;
    P=P0-delta_P;
    during:
    P=P0-delta_P;
    tv=t+t_s-t0;
  (default) -> work : {i=0; j=1; t0=0; t_s=t_start; P=1; tv=t_s;}
  work -> repair [order 1] : [P<=Pz]{i=i+1;t_s=0;}
  repair -> work : [t-t0>=delta_t]
  work -> repair [order 2] : [t+t_s>=trec*j]{j=j+1;t_s=0;i=0;}
  data: t_start input; delta_t input; Pz input; trec input; dP input; t input; tv output; P output; j local; delta_P local; t_s local; i local; t0 local; P0 input

== matlab function station_no_recovery/Восстанавливаемые объекты/УРАЛ-6000/Subsystem4/Element Normal/MATLAB Function ==
  data: t input; y output; sigma input; M input
function y = fcn(t,sigma,M)
y=normcdf((t-M)/sigma);

== stateflow chart station_no_recovery/Восстанавливаемые объекты/САТУРН/Subsystem1/Chart ==
  note: Параметры:
      | Входные:
      | dP - доля деградации при каждой итерации по вероятности
      | t - текущее время
      | Pz - заданная вероятность
      | P0 - вероятность, пересчитанная по времени
      | delta_t - время восстановления объекта
      | trec - время капитального ремонта
      | t_start - начальная выработка объекта
      |
      | Локальные:
      | i-количество восстановлений по вероятности(начинается с 0)
      | j-количество капитальных восстановлений (начинается с 1)
      | delta_P - dP * i
      | t0 - время, когда произошло восстановление (нужно для обнуления времени)
      | t_s = начальная выработка объекта (обнуляется после восстановления)
      |
      | Выходные:
      | tv - пересчитанное время
      | P - пересчитанная итоговая вероятность
  state repair
    entry:
    t0=t;
    tv=t-t0;
    P=0;
    during:
    P=0;
    tv=t-t0;
  state work
    entry:
    delta_P=dP*i;
    P=P0-delta_P;
    during:
    P=P0-delta_P;
    tv=t+t_s-t0;
  (default) -> work : {i=0; j=1; t0=0; t_s=t_start; P=1; tv=t_s;}
  work -> repair [order 1] : [P<=Pz]{i=i+1;t_s=0;}
  repair -> work : [t-t0>=delta_t]
  work -> repair [order 2] : [t+t_s>=trec*j]{j=j+1;t_s=0;i=0;}
  data: t_start input; delta_t input; Pz input; trec input; dP input; t input; tv output; P output; j local; delta_P local; t_s local; i local; t0 local; P0 input

== matlab function station_no_recovery/Восстанавливаемые объекты/САТУРН/Subsystem1/Element Normal/MATLAB Function ==
  data: t input; y output; sigma input; M input
function y = fcn(t,sigma,M)
y=normcdf((t-M)/sigma);

== stateflow chart station_no_recovery/Восстанавливаемые объекты/САТУРН/Subsystem2/Chart ==
  note: Параметры:
      | Входные:
      | dP - доля деградации при каждой итерации по вероятности
      | t - текущее время
      | Pz - заданная вероятность
      | P0 - вероятность, пересчитанная по времени
      | delta_t - время восстановления объекта
      | trec - время капитального ремонта
      | t_start - начальная выработка объекта
      |
      | Локальные:
      | i-количество восстановлений по вероятности(начинается с 0)
      | j-количество капитальных восстановлений (начинается с 1)
      | delta_P - dP * i
      | t0 - время, когда произошло восстановление (нужно для обнуления времени)
      | t_s = начальная выработка объекта (обнуляется после восстановления)
      |
      | Выходные:
      | tv - пересчитанное время
      | P - пересчитанная итоговая вероятность
  state repair
    entry:
    t0=t;
    tv=t-t0;
    P=0;
    during:
    P=0;
    tv=t-t0;
  state work
    entry:
    delta_P=dP*i;
    P=P0-delta_P;
    during:
    P=P0-delta_P;
    tv=t+t_s-t0;
  (default) -> work : {i=0; j=1; t0=0; t_s=t_start; P=1; tv=t_s;}
  work -> repair [order 1] : [P<=Pz]{i=i+1;t_s=0;}
  repair -> work : [t-t0>=delta_t]
  work -> repair [order 2] : [t+t_s>=trec*j]{j=j+1;t_s=0;i=0;}
  data: t_start input; delta_t input; Pz input; trec input; dP input; t input; tv output; P output; j local; delta_P local; t_s local; i local; t0 local; P0 input

== matlab function station_no_recovery/Восстанавливаемые объекты/САТУРН/Subsystem2/Element Normal/MATLAB Function ==
  data: t input; y output; sigma input; M input
function y = fcn(t,sigma,M)
y=normcdf((t-M)/sigma);

== stateflow chart station_no_recovery/Восстанавливаемые объекты/САТУРН/Subsystem3/Chart ==
  note: Параметры:
      | Входные:
      | dP - доля деградации при каждой итерации по вероятности
      | t - текущее время
      | Pz - заданная вероятность
      | P0 - вероятность, пересчитанная по времени
      | delta_t - время восстановления объекта
      | trec - время капитального ремонта
      | t_start - начальная выработка объекта
      |
      | Локальные:
      | i-количество восстановлений по вероятности(начинается с 0)
      | j-количество капитальных восстановлений (начинается с 1)
      | delta_P - dP * i
      | t0 - время, когда произошло восстановление (нужно для обнуления времени)
      | t_s = начальная выработка объекта (обнуляется после восстановления)
      |
      | Выходные:
      | tv - пересчитанное время
      | P - пересчитанная итоговая вероятность
  state repair
    entry:
    t0=t;
    tv=t-t0;
    P=0;
    during:
    P=0;
    tv=t-t0;
  state work
    entry:
    delta_P=dP*i;
    P=P0-delta_P;
    during:
    P=P0-delta_P;
    tv=t+t_s-t0;
  (default) -> work : {i=0; j=1; t0=0; t_s=t_start; P=1; tv=t_s;}
  work -> repair [order 1] : [P<=Pz]{i=i+1;t_s=0;}
  repair -> work : [t-t0>=delta_t]
  work -> repair [order 2] : [t+t_s>=trec*j]{j=j+1;t_s=0;i=0;}
  data: t_start input; delta_t input; Pz input; trec input; dP input; t input; tv output; P output; j local; delta_P local; t_s local; i local; t0 local; P0 input

== matlab function station_no_recovery/Восстанавливаемые объекты/САТУРН/Subsystem3/Element Normal/MATLAB Function ==
  data: t input; y output; sigma input; M input
function y = fcn(t,sigma,M)
y=normcdf((t-M)/sigma);

== stateflow chart station_no_recovery/Восстанавливаемые объекты/ГТЭ-6//6,3/Subsystem2/Chart ==
  note: Параметры:
      | Входные:
      | dP - доля деградации при каждой итерации по вероятности
      | t - текущее время
      | Pz - заданная вероятность
      | P0 - вероятность, пересчитанная по времени
      | delta_t - время восстановления объекта
      | trec - время капитального ремонта
      | t_start - начальная выработка объекта
      |
      | Локальные:
      | i-количество восстановлений по вероятности(начинается с 0)
      | j-количество капитальных восстановлений (начинается с 1)
      | delta_P - dP * i
      | t0 - время, когда произошло восстановление (нужно для обнуления времени)
      | t_s = начальная выработка объекта (обнуляется после восстановления)
      |
      | Выходные:
      | tv - пересчитанное время
      | P - пересчитанная итоговая вероятность
  state repair
    entry:
    t0=t;
    tv=t-t0;
    P=0;
    during:
    P=0;
    tv=t-t0;
  state work
    entry:
    delta_P=dP*i;
    P=P0-delta_P;
    during:
    P=P0-delta_P;
    tv=t+t_s-t0;
  (default) -> work : {i=0; j=1; t0=0; t_s=t_start; P=1; tv=t_s;}
  work -> repair [order 1] : [P<=Pz]{i=i+1;t_s=0;}
  repair -> work : [t-t0>=delta_t]
  work -> repair [order 2] : [t+t_s>=trec*j]{j=j+1;t_s=0;i=0;}
  data: t_start input; delta_t input; Pz input; trec input; dP input; t input; tv output; P output; j local; delta_P local; t_s local; i local; t0 local; P0 input

== matlab function station_no_recovery/Восстанавливаемые объекты/ГТЭ-6//6,3/Subsystem2/Element Normal/MATLAB Function ==
  data: t input; y output; sigma input; M input
function y = fcn(t,sigma,M)
y=normcdf((t-M)/sigma);

== stateflow chart station_no_recovery/Восстанавливаемые объекты/ЭГ-12/Subsystem1/Chart ==
  note: Параметры:
      | Входные:
      | dP - доля деградации при каждой итерации по вероятности
      | t - текущее время
      | Pz - заданная вероятность
      | P0 - вероятность, пересчитанная по времени
      | delta_t - время восстановления объекта
      | trec - время капитального ремонта
      | t_start - начальная выработка объекта
      |
      | Локальные:
      | i-количество восстановлений по вероятности(начинается с 0)
      | j-количество капитальных восстановлений (начинается с 1)
      | delta_P - dP * i
      | t0 - время, когда произошло восстановление (нужно для обнуления времени)
      | t_s = начальная выработка объекта (обнуляется после восстановления)
      |
      | Выходные:
      | tv - пересчитанное время
      | P - пересчитанная итоговая вероятность
  state repair
    entry:
    t0=t;
    tv=t-t0;
    P=0;
    during:
    P=0;
    tv=t-t0;
  state work
    entry:
    delta_P=dP*i;
    P=P0-delta_P;
    during:
    P=P0-delta_P;
    tv=t+t_s-t0;
  (default) -> work : {i=0; j=1; t0=0; t_s=t_start; P=1; tv=t_s;}
  work -> repair [order 1] : [P<=Pz]{i=i+1;t_s=0;}
  repair -> work : [t-t0>=delta_t]
  work -> repair [order 2] : [t+t_s>=trec*j]{j=j+1;t_s=0;i=0;}
  data: t_start input; delta_t input; Pz input; trec input; dP input; t input; tv output; P output; j local; delta_P local; t_s local; i local; t0 local; P0 input

== matlab function station_no_recovery/Восстанавливаемые объекты/ЭГ-12/Subsystem1/Element Normal/MATLAB Function ==
  data: t input; y output; sigma input; M input
function y = fcn(t,sigma,M)
y=normcdf((t-M)/sigma);

== matlab function station_no_recovery/Схема/Сircuit n Parallel2/n Parallel Function ==
  data: Pn output; P input
function Pn = fcn(P)
[n,col]=size(P);
u=1;
for i=1:n
   u=u*(1-P(i)); 
end
Pn = 1 - u;

== matlab function station_no_recovery/Схема/Сircuit n Parallel3/n Parallel Function ==
  data: Pn output; P input
function Pn = fcn(P)
[n,col]=size(P);
u=1;
for i=1:n
   u=u*(1-P(i)); 
end
Pn = 1 - u;

== matlab function station_no_recovery/Схема/Сircuit n Parallel4/n Parallel Function ==
  data: Pn output; P input
function Pn = fcn(P)
[n,col]=size(P);
u=1;
for i=1:n
   u=u*(1-P(i)); 
end
Pn = 1 - u;

== matlab function station_no_recovery/Схема/Сircuit n Parallel5/n Parallel Function ==
  data: Pn output; P input
function Pn = fcn(P)
[n,col]=size(P);
u=1;
for i=1:n
   u=u*(1-P(i)); 
end
Pn = 1 - u;

== matlab function station_no_recovery/Схема/Сircuit n Series5/n Series Function ==
  data: Pn output; P input
function Pn = fcn(P)
[n,col]=size(P);
u=1;
for i=1:n
   u=u*P(i); 
end
Pn = u;

== matlab function station_no_recovery/Схема/Сircuit n Series6/n Series Function ==
  data: Pn output; P input
function Pn = fcn(P)
[n,col]=size(P);
u=1;
for i=1:n
   u=u*P(i); 
end
Pn = u;

== matlab function station_no_recovery/Схема/Сircuit n Series7/n Series Function ==
  data: Pn output; P input
function Pn = fcn(P)
[n,col]=size(P);
u=1;
for i=1:n
   u=u*P(i); 
end
Pn = u;

== matlab function station_no_recovery/Схема/Сircuit n Series8/n Series Function ==
  data: Pn output; P input
function Pn = fcn(P)
[n,col]=size(P);
u=1;
for i=1:n
   u=u*P(i); 
end
Pn = u;

== matlab function station_no_recovery/Схема/Сircuit Bridge2/parallel circuit 1-2 4-5 1-3-5 4-3-2/n Parallel Function ==
  data: Pn output; P input
function Pn = fcn(P)
[n,col]=size(P);
u=1;
for i=1:n
   u=u*(1-P(i)); 
end

Pn = 1 - u;

== matlab function station_no_recovery/Схема/Сircuit Bridge2/series circuit 1, 3, 5/n Series Function ==
  data: Pn output; P input
function Pn = fcn(P)
[n,col]=size(P);
u=1;
for i=1:n
   u=u*P(i); 
end

Pn = u;

== matlab function station_no_recovery/Схема/Сircuit Bridge2/series circuit 4, 3, 2/n Series Function ==
  data: Pn output; P input
function Pn = fcn(P)
[n,col]=size(P);
u=1;
for i=1:n
   u=u*P(i); 
end

Pn = u;
